simulink library "foc_ltid_blocks"  (R2024b)
settings: Solver=VariableStepAuto  StartTime=0.0  StopTime=10.0  RelTol=1e-3
settings Model: Creator=ZONG CHUHANG  LastModifiedBy=ZONG CHUHANG

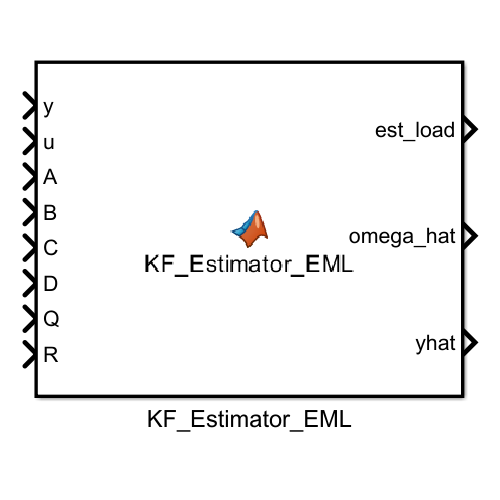
[thumbnail: Simulink's stored preview of the top-level diagram]
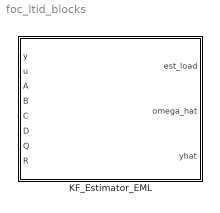
== system foc_ltid_blocks ==
  KF_Estimator_EML : MATLAB Function  TreatAsAtomicUnit=on

== matlab function foc_ltid_blocks/KF_Estimator_EML ==
  data: y input; u input; est_load output; A input; B input; C input; D input; Q input; R input; omega_hat output; yhat output
function [est_load, omega_hat, yhat] = KF_Estimator_EML(y, u, A, B, C, D, Q, R)
%#codegen
% Generic discrete observer / Kalman-filter recursion (shared formula F6.a).
% Reduces to a fixed-gain Luenberger observer (F4/F5) when driven by a constant gain.
% State convention (shared formula F2): x = [omega_m ; T_load], u = Te, y = omega_m.
% A,B,C,D,Q,R arrive as inputs (wire Constants sourced from InitFcn workspace vars);
% this atom holds NO numeric values of its own.
persistent xhat P
n = size(A,1);
if isempty(xhat)
    xhat = zeros(n,1);
    P    = eye(n);
end
% --- time update (predict) ---
xhat = A*xhat + B*u;
P    = A*P*A.' + Q;
% --- measurement update (correct) ---
S     = C*P*C.' + R;
K     = (P*C.') / S;
resid = y - (C*xhat + D*u);
xhat  = xhat + K*resid;
P     = (eye(n) - K*C)*P;
% --- outputs ---
omega_hat = xhat(1);
est_load  = xhat(2);   % load-torque estimate (F2 state 2) -> F8 feed-forward
yhat      = C*xhat + D*u;
end
